simulink model "J542"  (R2015b)
settings: Solver=VariableStepAuto  StartTime=-10  StopTime=10.0  RelTol=1e-3
libraries: simulink x1
settings Model: Creator=Pouya  LastModifiedBy=Pouya

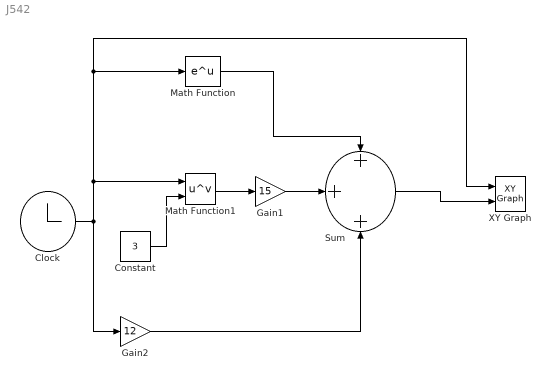
== system J542 ==
  Clock : Clock
  Constant : Constant  Value=3
  Gain1 : Gain  Gain=15
  Gain2 : Gain  Gain=12
  Math Function : Math  SaturateOnIntegerOverflow=on
  Math Function1 : Math  Operator=pow  SaturateOnIntegerOverflow=on
  Sum : Sum  Inputs=+++
  XY Graph : simulink/Sinks/XY Graph  xmin=-10  xmax=10  ymin=-100  ymax=100  st=-1
  wires:
  Clock/1 -> Math Function1/1, Math Function/1, XY Graph/1, Gain2/1
  Constant/1 -> Math Function1/2
  Math Function/1 -> Sum/1
  Gain2/1 -> Sum/3
  Sum/1 -> XY Graph/2
  Math Function1/1 -> Gain1/1
  Gain1/1 -> Sum/2
